simulink model "Autonomous_Driving"  (R2021a)
settings: Solver=ode2  StartTime=0.0  StopTime=inf  FixedStep=1/600  RelTol=1e-3  EnableMultiTasking=on
model workspace (MAT data in the model file):
  camera_rate : Simulink.Parameter (value not decoded)
  depth_rate : Simulink.Parameter (value not decoded)
symbols that are objects in the model workspace (value not decoded): camera_rate, depth_rate
undefined symbols (not defined in the file): gcbh, HIL, JPEG, qc_get_step_size, Video3D, video_display_show
libraries: quarc_library x32, simulink x15
(part 2 of 2)

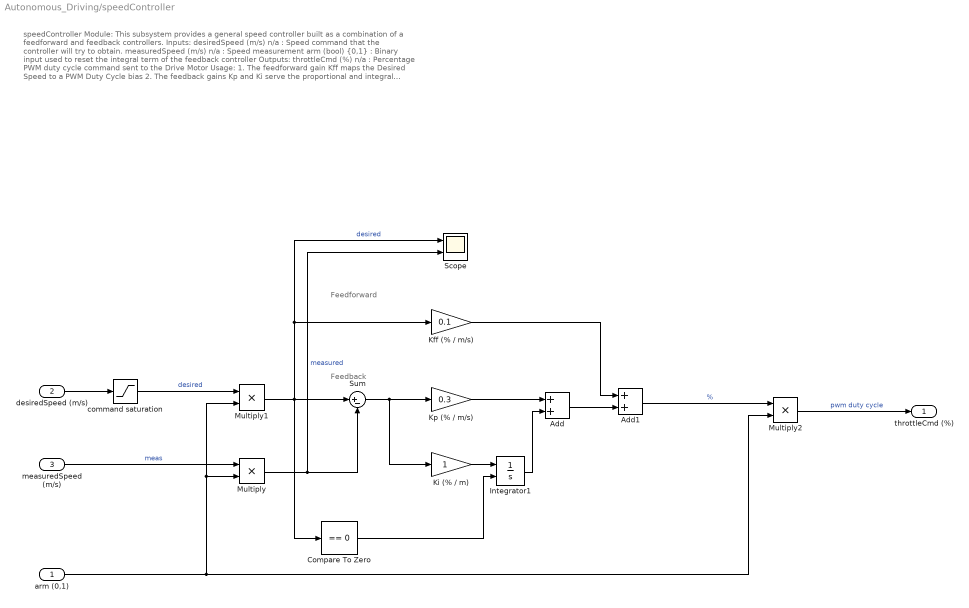
== system Autonomous_Driving/speedController ==
  note: Feedforward
  note: Feedback
  note: speedController Module:
      |
      | This subsystem provides a general speed controller built as a combination of a feedforward and feedback controllers.
      |
      | Inputs:
      | desiredSpeed (m/s) n/a : Speed command that the controller will try to obtain.
      | measuredSpeed (m/s) n/a : Speed measurement
      | arm (bool) {0,1} : Binary input used to reset the integral term of the feedback controller
      |
      | Outputs:
      | throttleCmd (%) n/a : Percentage PWM duty cycle command sent to the Drive Motor
      |
      | Usage:
      | 1. The feedforward gain Kff maps the Desired Speed to a PWM Duty Cycle bias
      | 2. The feedback gains Kp and Ki serve the proportional and integral terms to output corrections to the PWM Duty Cycle so as to regulate the desired speed.
  arm (0,1) : Inport
  desiredSpeed (m/s) : Inport  Port=2
  measuredSpeed (m/s) : Inport  Port=3
  Add : Sum
  Add1 : Sum
  Compare To Zero : simulink/Logic and Bit Operations/Compare To Zero  relop===  OutDataTypeStr=boolean
  Integrator1 : Integrator  ExternalReset=either  LimitOutput=on  UpperSaturationLimit=0.4  LowerSaturationLimit=-0.4
  Kff (% / m/s) : Gain  Gain=0.1
  "Ki (% / m) " : Gain
  Kp (% / m/s) : Gain  Gain=0.3
  Multiply : Product
  Multiply1 : Product
  Multiply2 : Product
  Scope : Scope  NumInputPorts=2
  Sum : Sum  Inputs=|+-
  command saturation : Saturate  UpperLimit=5  LowerLimit=-5
  throttleCmd (%) : Outport  VectorParamsAs1DForOutWhenUnconnected=off
  wires:
  command saturation/1 -> Multiply1/1  "desired"
  arm (0,1)/1 -> Multiply1/2, Multiply/2, Multiply2/2
  measuredSpeed (m/s)/1 -> Multiply/1  "meas"
  Multiply/1 -> Sum/2, Scope/2  "measured"
  Add/1 -> Add1/2
  Add1/1 -> Multiply2/1  "%"
  Multiply1/1 -> Compare To Zero/1, Sum/1, Kff (% / m/s)/1, Scope/1  "desired"
  Integrator1/1 -> Add/2
  Multiply2/1 -> throttleCmd (%)/1  "pwm duty cycle"
  Kp (% / m/s)/1 -> Add/1
  Compare To Zero/1 -> Integrator1/2
  Kff (% / m/s)/1 -> Add1/1
  Sum/1 -> "Ki (% / m) "/1, Kp (% / m/s)/1
  "Ki (% / m) "/1 -> Integrator1/1
  desiredSpeed (m/s)/1 -> command saturation/1

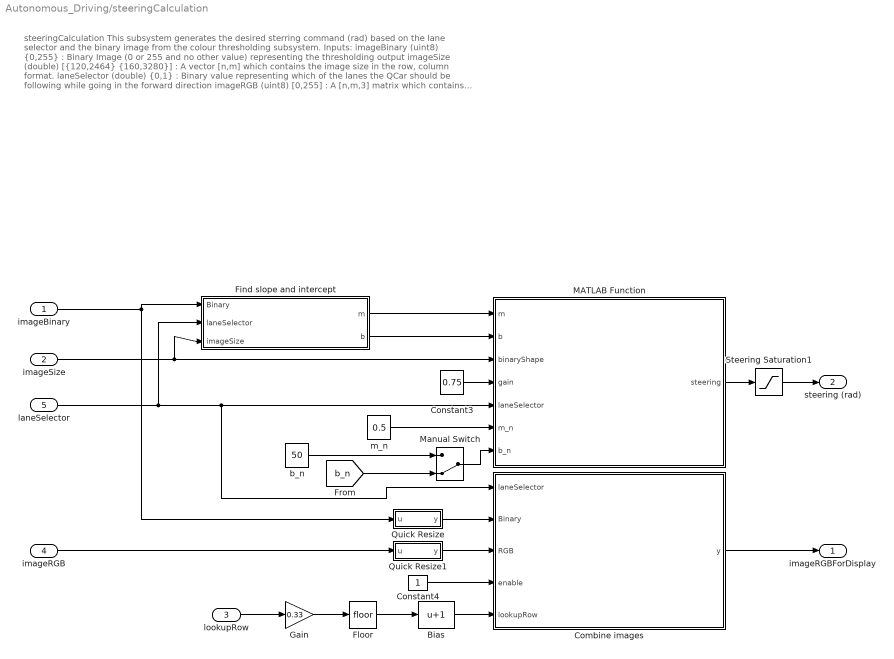
== system Autonomous_Driving/steeringCalculation ==
  note: steeringCalculation
      | This subsystem generates the desired sterring command (rad) based on the lane selector and the binary image from the colour thresholding subsystem.
      |
      | Inputs:
      | imageBinary (uint8) {0,255} : Binary Image (0 or 255 and no other value) representing the thresholding output
      | imageSize (double) [{120,2464} {160,3280}] : A vector [n,m] which contains the image size in the row, column format.
      | laneSelector (double) {0,1} : Binary value representing which of the lanes the QCar should be following while going in the forward direction
      | imageRGB (uint8) [0,255] : A [n,m,3] matrix which contains RGB values of an image in uint8 format
      |
      | Outputs:
      | steering (double) {-0.5,0.5} : Angle in rad representing the desired steering command based on the linearPolyFit
      | imageRGBForDisplay (uint8) {0,255} : A [n,m,3] matrix representing an RGB Image with mask of the lane currently being tracked
      |
      | Usage:
      |
      | This module can be used to generate a desired steering angle based on a thresheld image. A linear polygonal fit is used to generate a slope based on the equation y = mx+b whose slope and y intercept will define the steering angle commanded up to 0.5 (rad). The RGB image is a combination of the binary image holding information of the lane being followed, and a scaled version of the original RGB image.
  imageBinary : Inport
  imageSize : Inport  Port=2
  lookupRow : Inport  Port=3
  imageRGB : Inport  Port=4
  laneSelector : Inport  Port=5
  Bias : Bias  Bias=1
  Combine images : MATLAB Function  TreatAsAtomicUnit=on
  Constant3 : Constant  Value=0.75
  Constant4 : Constant
  Find slope and intercept : MATLAB Function  TreatAsAtomicUnit=on
  Floor : Rounding
  Gain : Gain  Gain=0.33
  MATLAB Function : MATLAB Function  TreatAsAtomicUnit=on
  Manual Switch : ManualSwitch  CurrentSetting=0
  Quick Resize : MATLAB Function  TreatAsAtomicUnit=on
  Quick Resize1 : MATLAB Function  TreatAsAtomicUnit=on
  Steering Saturation1 : Saturate
  b_n : Constant  Value=50
  m_n : Constant  Value=0.5
  imageRGBForDisplay : Outport  VectorParamsAs1DForOutWhenUnconnected=off
  steering (rad) : Outport  Port=2  VectorParamsAs1DForOutWhenUnconnected=off
  wires:
  Find slope and intercept/1(m) -> MATLAB Function/1(m)
  laneSelector/1 -> MATLAB Function/5(laneSelector), Combine images/1(laneSelector), Find slope and intercept/2(laneSelector)
  MATLAB Function/1(steering) -> Steering Saturation1/1
  Constant3/1 -> MATLAB Function/4(gain)
  imageBinary/1 -> Quick Resize/1(u), Find slope and intercept/1(Binary)
  Find slope and intercept/2(b) -> MATLAB Function/2(b)
  Constant4/1 -> Combine images/4(enable)
  Quick Resize/1(y) -> Combine images/2(Binary)
  Quick Resize1/1(y) -> Combine images/3(RGB)
  Combine images/1(y) -> imageRGBForDisplay/1
  imageRGB/1 -> Quick Resize1/1(u)
  Steering Saturation1/1 -> steering (rad)/1
  Gain/1 -> Floor/1
  imageSize/1 -> Find slope and intercept/3(imageSize), MATLAB Function/3(binaryShape)
  lookupRow/1 -> Gain/1
  Bias/1 -> Combine images/5(lookupRow)
  Floor/1 -> Bias/1
  b_n/1 -> Manual Switch/1
  Manual Switch/1 -> MATLAB Function/7(b_n)
  [b_n] -> Manual Switch/2
  m_n/1 -> MATLAB Function/6(m_n)

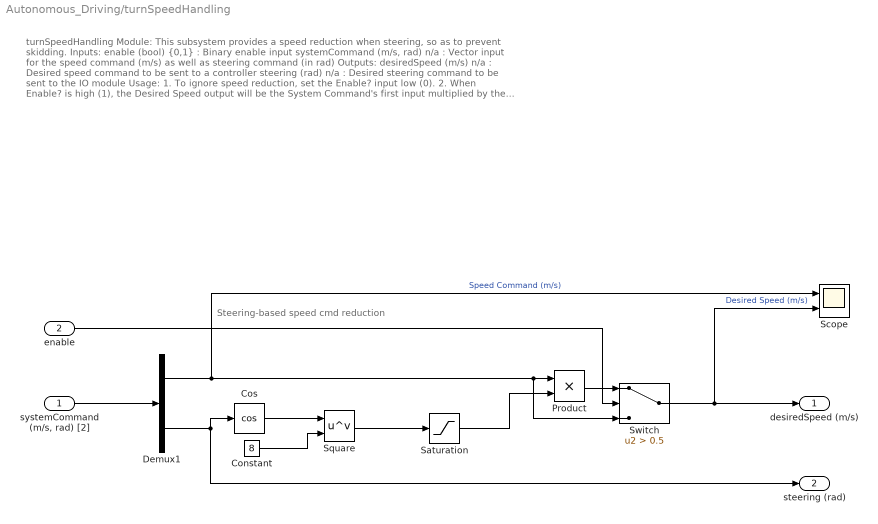
== system Autonomous_Driving/turnSpeedHandling ==
  note: turnSpeedHandling Module:
      |
      | This subsystem provides a speed reduction when steering, so as to prevent skidding.
      |
      | Inputs:
      | enable (bool) {0,1} : Binary enable input
      | systemCommand (m/s, rad) n/a : Vector input for the speed command (m/s) as well as steering command (in rad)
      |
      | Outputs:
      | desiredSpeed (m/s) n/a : Desired speed command to be sent to a controller
      | steering (rad) n/a : Desired steering command to be sent to the IO module
      |
      | Usage:
      | 1. To ignore speed reduction, set the Enable? input low (0).
      | 2. When Enable? is high (1), the Desired Speed output will be the System Command's first input multiplied by the cosine of the steering. Note that the lower limit of this reduction is set to 50% of the speed command input.
  note: Steering-based speed cmd reduction
  "systemCommand (m/s, rad) [2]" : Inport
  enable : Inport  Port=2
  Constant : Constant  Value=8
  Cos : Trigonometry  Operator=cos
  Demux1 : Demux  Outputs=2
  Product : Product
  Saturation : Saturate  UpperLimit=1  LowerLimit=0.5
  Scope : Scope  NumInputPorts=2
  Square : Math  Operator=pow  SignedPower=on  SaturateOnIntegerOverflow=on
  Switch : Switch  Criteria=u2 > Threshold  Threshold=0.5
  desiredSpeed (m/s) : Outport  VectorParamsAs1DForOutWhenUnconnected=off
  steering (rad) : Outport  Port=2  VectorParamsAs1DForOutWhenUnconnected=off
  wires:
  Cos/1 -> Square/1
  Switch/1 -> desiredSpeed (m/s)/1, Scope/2  "Desired Speed (m/s)"
  Product/1 -> Switch/1
  Saturation/1 -> Product/2
  Demux1/1 -> Product/1, Switch/3, Scope/1  "Speed Command (m/s)"
  "systemCommand (m/s, rad) [2]"/1 -> Demux1/1
  enable/1 -> Switch/2
  Constant/1 -> Square/2
  Demux1/2 -> steering (rad)/1, Cos/1
  Square/1 -> Saturation/1

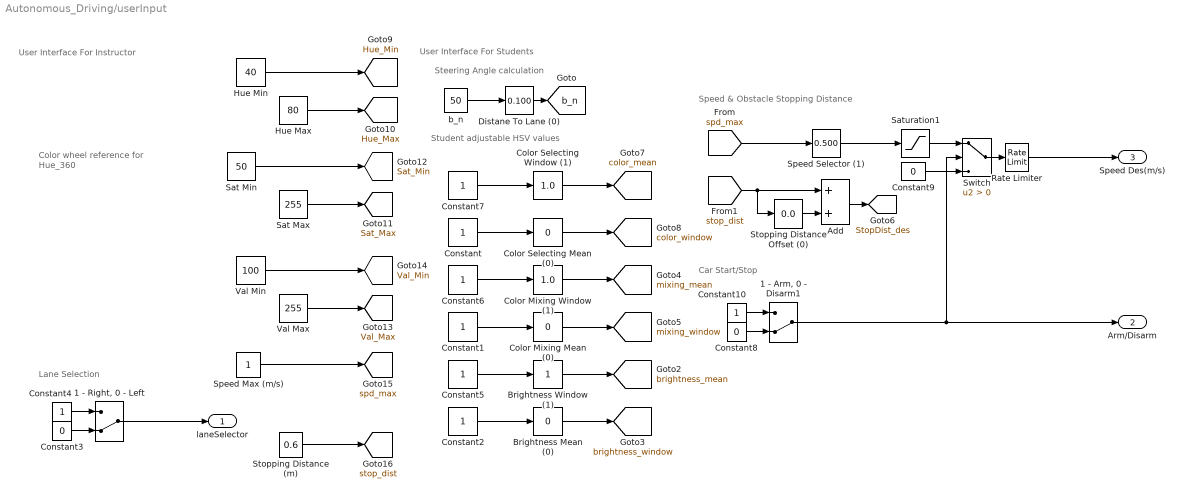
== system Autonomous_Driving/userInput ==
  note: User Interface For Instructor
  note: Student adjustable HSV values
  note: Lane Selection
  note: Car Start/Stop
  note: Steering Angle calculation
  note: User Interface For Students
  note: Speed & Obstacle Stopping Distance
  note: Color wheel
      | reference
      | for Hue_360
  "1 - Arm, 0 - Disarm1" : ManualSwitch  CurrentSetting=0
  "1 - Right, 0 - Left" : ManualSwitch  CurrentSetting=0
  Add : Sum
  Brightness Mean (0) : simulink/Math Operations/Slider Gain  gain=0  low=-1  high=1
  Brightness Window (1) : simulink/Math Operations/Slider Gain  gain=1  low=0  high=1
  Color Mixing Mean (0) : simulink/Math Operations/Slider Gain  gain=0  low=-1  high=1
  Color Mixing Window (1) : simulink/Math Operations/Slider Gain  gain=1.0  low=0  high=1
  Color Selecting Mean (0) : simulink/Math Operations/Slider Gain  gain=0  low=-1  high=1
  Color Selecting Window (1) : simulink/Math Operations/Slider Gain  gain=1.0  low=0  high=1
  Constant{,1..2,4..7,10} (8 alike) : Constant
  Constant3 : Constant  Value=0
  Constant8 : Constant  Value=0
  Constant9 : Constant  Value=0
  "Distane To Lane (0) " : simulink/Math Operations/Slider Gain  gain=0.100  low=0  high=1
  Hue Max : Constant  Value=80
  Hue Min : Constant  Value=40
  Rate Limiter : RateLimiter  FallingSlewLimit=-Inf  SampleTimeMode=inherited
  Sat Max : Constant  Value=255
  Sat Min : Constant  Value=50
  Saturation1 : Saturate  UpperLimit=1  LowerLimit=0
  Speed Max (m/s) : Constant
  Speed Selector (1) : simulink/Math Operations/Slider Gain  gain=0.500  low=0  high=1
  Stopping Distance (m) : Constant  Value=0.6
  Stopping Distance Offset (0) : simulink/Math Operations/Slider Gain  gain=0.0  low=0  high=1
  Switch : Switch  Criteria=u2 > Threshold
  Val Max : Constant  Value=255
  Val Min : Constant  Value=100
  b_n : Constant  Value=50
  laneSelector : Outport  VectorParamsAs1DForOutWhenUnconnected=off
  Arm/Disarm : Outport  Port=2  VectorParamsAs1DForOutWhenUnconnected=off
  Speed Des(m/s) : Outport  Port=3  VectorParamsAs1DForOutWhenUnconnected=off
  tag scope: Hue_Max=global, Hue_Min=global, Sat_Max=global, Sat_Min=global, StopDist_des=global, Val_Max=global, Val_Min=global, b_n=global, brightness_mean=global, brightness_window=global, color_mean=global, color_window=global, mixing_mean=global, mixing_window=global, spd_max=global, stop_dist=global
  wires:
  Constant3/1 -> "1 - Right, 0 - Left"/2
  "1 - Arm, 0 - Disarm1"/1 -> Switch/2, Arm/Disarm/1
  b_n/1 -> "Distane To Lane (0) "/1
  Constant4/1 -> "1 - Right, 0 - Left"/1
  Switch/1 -> Rate Limiter/1
  Constant9/1 -> Switch/3
  [spd_max] -> Speed Selector (1)/1
  Saturation1/1 -> Switch/1
  Constant10/1 -> "1 - Arm, 0 - Disarm1"/1
  "1 - Right, 0 - Left"/1 -> laneSelector/1
  Rate Limiter/1 -> Speed Des(m/s)/1
  Constant8/1 -> "1 - Arm, 0 - Disarm1"/2
  "Distane To Lane (0) "/1 -> [b_n]
  Color Mixing Window (1)/1 -> [mixing_mean]
  Constant/1 -> Color Selecting Mean (0)/1
  Constant2/1 -> Brightness Mean (0)/1
  Constant5/1 -> Brightness Window (1)/1
  Constant1/1 -> Color Mixing Mean (0)/1
  Color Selecting Mean (0)/1 -> [color_window]
  Brightness Window (1)/1 -> [brightness_mean]
  Color Selecting Window (1)/1 -> [color_mean]
  Brightness Mean (0)/1 -> [brightness_window]
  Color Mixing Mean (0)/1 -> [mixing_window]
  Constant6/1 -> Color Mixing Window (1)/1
  Constant7/1 -> Color Selecting Window (1)/1
  Hue Min/1 -> [Hue_Min]
  Sat Min/1 -> [Sat_Min]
  Val Min/1 -> [Val_Min]
  Hue Max/1 -> [Hue_Max]
  Sat Max/1 -> [Sat_Max]
  Val Max/1 -> [Val_Max]
  Speed Selector (1)/1 -> Saturation1/1
  Speed Max (m/s)/1 -> [spd_max]
  Stopping Distance (m)/1 -> [stop_dist]
  [stop_dist] -> Stopping Distance Offset (0)/1, Add/1
  Stopping Distance Offset (0)/1 -> Add/2
  Add/1 -> [StopDist_des]

== system Autonomous_Driving/Display Depth/Depth Camera Information ==
  In1 : Inport
  Channel : quarc_library/Signal Routing/Channel  channel=0  buffer_size=1
  Image Compress : quarc_library/Image Processing/Generic/Image Compress  algorithm=JPEG  source=Internal dialog parameter  quality=quality  output_dim=-1
  Video Display : quarc_library/Multimedia/Video Display  Tag=Autonomous_Driving/Display Depth/Depth Camera Information/Video Display  sample_time=sample_time  use_hardware=on
  wires:
  Image Compress/1 -> Channel/1
  In1/1 -> Image Compress/1
  Channel/1 -> Video Display/1

== system Autonomous_Driving/Display RGB/RGB Image Processed ==
  In1 : Inport
  Channel : quarc_library/Signal Routing/Channel  channel=1  buffer_size=1
  Image Compress : quarc_library/Image Processing/Generic/Image Compress  algorithm=JPEG  source=Internal dialog parameter  quality=quality  output_dim=-1
  Video Display : quarc_library/Multimedia/Video Display  Tag=Autonomous_Driving/Display RGB/RGB Image Processed/Video Display  sample_time=sample_time  use_hardware=on
  wires:
  Image Compress/1 -> Channel/1
  In1/1 -> Image Compress/1
  Channel/1 -> Video Display/1

== system Autonomous_Driving/RGB Image Pre-Proccessing/RGB Image No Threshold ==
  In1 : Inport
  Channel : quarc_library/Signal Routing/Channel  channel=2  buffer_size=1
  Image Compress : quarc_library/Image Processing/Generic/Image Compress  algorithm=JPEG  source=Internal dialog parameter  quality=quality  output_dim=-1
  Video Display : quarc_library/Multimedia/Video Display  Tag="Autonomous_Driving/RGB Image  Pre-Proccessing/RGB Image No Threshold/Video Display"  sample_time=sample_time  use_hardware=on
  wires:
  Channel/1 -> Video Display/1
  In1/1 -> Image Compress/1
  Image Compress/1 -> Channel/1

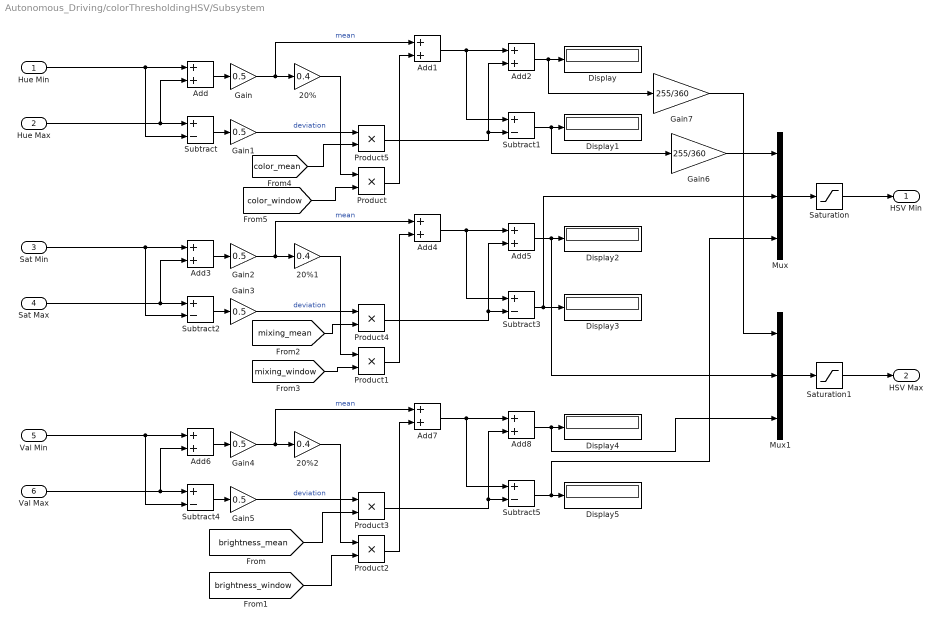
== system Autonomous_Driving/colorThresholdingHSV/Subsystem ==
  Hue Min : Inport
  Hue Max : Inport  Port=2
  Sat Min : Inport  Port=3
  Sat Max : Inport  Port=4
  Val Min : Inport  Port=5
  Val Max : Inport  Port=6
  20% : Gain  Gain=0.4
  20%1 : Gain  Gain=0.4
  20%2 : Gain  Gain=0.4
  Add{,1..8} (9 alike) : Sum
  Display{,1..5} (6 alike) : Display
  Gain{,1..5} (6 alike) : Gain  Gain=0.5
  Gain6 : Gain  Gain=255/360
  Gain7 : Gain  Gain=255/360
  Mux : Mux  Inputs=3
  Mux1 : Mux  Inputs=3
  Product{,1..5} (6 alike) : Product
  Saturation : Saturate  UpperLimit=[255 255 255]  LowerLimit=[0 0 0]
  Saturation1 : Saturate  UpperLimit=[255 255 255]  LowerLimit=[0 0 0]
  Subtract{,1..5} (6 alike) : Sum  Inputs=+-
  HSV Min : Outport  VectorParamsAs1DForOutWhenUnconnected=off
  HSV Max : Outport  Port=2  VectorParamsAs1DForOutWhenUnconnected=off
  wires:
  Product1/1 -> Add4/2
  Val Min/1 -> Add6/1, Subtract4/2
  Mux/1 -> Saturation/1
  Subtract1/1 -> Gain6/1, Display1/1
  Subtract4/1 -> Gain5/1
  Add1/1 -> Subtract1/1, Add2/1
  Product3/1 -> Add8/2, Subtract5/2
  Product2/1 -> Add7/2
  Gain4/1 -> 20%2/1, Add7/1  "mean"
  Add2/1 -> Gain7/1, Display/1
  Subtract3/1 -> Mux/2, Display3/1
  Subtract5/1 -> Mux/3, Display5/1
  Gain/1 -> 20%/1, Add1/1  "mean"
  Sat Min/1 -> Subtract2/2, Add3/1
  Subtract2/1 -> Gain3/1
  Product5/1 -> Add2/2, Subtract1/2
  Gain5/1 -> Product3/1  "deviation"
  Add5/1 -> Mux1/2, Display2/1
  Gain2/1 -> Add4/1, 20%1/1  "mean"
  Add8/1 -> Mux1/3, Display4/1
  Product/1 -> Add1/2
  Subtract/1 -> Gain1/1
  Product4/1 -> Subtract3/2, Add5/2
  Add4/1 -> Add5/1, Subtract3/1
  Add7/1 -> Subtract5/1, Add8/1
  Sat Max/1 -> Subtract2/1, Add3/2
  20%1/1 -> Product1/1
  [brightness_mean] -> Product3/2
  Mux1/1 -> Saturation1/1
  Add3/1 -> Gain2/1
  [mixing_mean] -> Product4/2
  Hue Min/1 -> Add/1, Subtract/2
  Hue Max/1 -> Add/2, Subtract/1
  Gain3/1 -> Product4/1  "deviation"
  Val Max/1 -> Add6/2, Subtract4/1
  20%2/1 -> Product2/1
  Add6/1 -> Gain4/1
  [color_window] -> Product/2
  [color_mean] -> Product5/2
  20%/1 -> Product/1
  Add/1 -> Gain/1
  Gain1/1 -> Product5/1  "deviation"
  [mixing_window] -> Product1/2
  [brightness_window] -> Product2/2
  Saturation/1 -> HSV Min/1
  Saturation1/1 -> HSV Max/1
  Gain6/1 -> Mux/1
  Gain7/1 -> Mux1/1

== matlab function Autonomous_Driving/MATLAB Function ==
  data: imageRGB input; imageToThreshold output; laneSelector input; lookupRow input; imageSize output
function [imageToThreshold, imageSize]  = imageSelector(imageRGB, laneSelector, lookupRow)

[ROW, COL, ~] = size(imageRGB);
% imageToThreshold = uint8(zeros(ROW/2+1,COL/3,3));
if laneSelector
    imageToThreshold = imageRGB(ROW/2+1:ROW, COL*(2/3) + 1:COL, :);
else
    imageToThreshold = imageRGB(ROW/2+1:ROW, 1:COL/3, :);
end
imageToThreshold(1: ROW/2 - (ROW - lookupRow + 1),:,:) = 0;
imageSize = [ROW - lookupRow + 1, COL/3];

== matlab function Autonomous_Driving/obstacleDetection/Draw Lines Module ==
  data: img_in input; img_out output; pts input; color input
function img_out = drawLines(img_in, pts, color)

% Draw lines connecting the points using the provided color

% Inputs:
% img_in    : Input RGB Image (size = m by n)
% pts       : p x-y pairs of points (px) where markers are to be drawn
% color     : 1x3 matrix of RGB color values for each marker

% Outputs:
% img_out   : Output RGB Image with the markers drawn in (size = m by n)

%% Initialization
if size(img_in, 3) == 3
    img_out = img_in;
elseif size(img_in, 3) == 1
    img_out = cat(3, img_in, img_in, img_in);
end

[p, ~] = size(pts); % determine the number of points

%% Draw the lines
    for i = 1:p-1
        % determine the max(rows_difference, col_difference) between two
        % points
        itr = max(abs(pts(i,1) - pts(i+1,1)), abs(pts(i,2) - pts(i+1,2)));
        
        % generate linear spaces of row and col values between the pts
        row_vec = round(linspace(pts(i,1), pts(i+1,1), itr));
        col_vec = round(linspace(pts(i,2), pts(i+1,2), itr));
        
        % iterate through the values and shade them right

        for j = 1:itr
            img_out(row_vec(j), col_vec(j),1) = color(1);
            img_out(row_vec(j), col_vec(j),2) = color(2);
            img_out(row_vec(j), col_vec(j),3) = color(3);
        end
    end
end

== matlab function Autonomous_Driving/steeringCalculation/Find slope and intercept ==
  data: Binary input; m output; b output; laneSelector input; imageSize input
function [m, b] = linearPolyFit(Binary, laneSelector, imageSize)

% find the shape of the incoming image
[ROW, ~] = size(Binary);

% find row, col pairs of points where pixel value is bright
[rows, cols] = find(Binary(ROW - imageSize(1) + 1:end, :) > 0);

% x is coloumns, y is max_row - rows
if laneSelector
    x = imageSize(2) - cols;
else
    x = cols;
end

y = imageSize(1) - rows;

% fit a linear polynomial to the points and grab slope, intercept
% result = polyfit(x(idx), y(idx), 1);
result = polyfit(x, y, 1);
m = result(1); 
b = result(2);

== matlab function Autonomous_Driving/steeringCalculation/MATLAB Function ==
  data: m input; steering output; b input; binaryShape input; gain input; laneSelector input; m_n input; b_n input
function steering = fcn(m, b, binaryShape, gain, laneSelector, m_n, b_n)
 
% y = mx + b

current_x = (binaryShape(1) - b)/m;
nominal_x = (binaryShape(1) - b_n)/m_n;
if laneSelector
    steering = -gain*(nominal_x - current_x)/binaryShape(2);
else
    steering = gain*(nominal_x - current_x)/binaryShape(2);
end

== matlab function Autonomous_Driving/steeringCalculation/Quick Resize ==
  data: u input; y output
function y = quickResize(u)

scale = 3;
    if length(size(u)) == 3
        y = u(1:scale:end, 1:scale:end, :);
    else
        y = u(1:scale:end, 1:scale:end);
    end

end

== matlab function Autonomous_Driving/steeringCalculation/Combine images ==
  data: laneSelector input; Binary input; RGB input; y output size=[137,274,3]; enable input; lookupRow input
function y = laneMask(laneSelector, Binary, RGB, enable, lookupRow)

y = RGB;
[ROW, COL, ~] = size(y);
[binRow, ~] = size(Binary);
binarySection = Binary(binRow-(length(lookupRow:ROW))+1:binRow,:);
if enable
    if laneSelector
        section = RGB(lookupRow:ROW, COL*(2/3) + 1:COL, :);
        y(lookupRow:ROW, COL*(2/3) + 1:COL, 1) = ((255 - binarySection)/255).*section(:,:,1) + (binarySection).*section(:, :, 1);
        y(lookupRow:ROW, COL*(2/3) + 1:COL, 2) = ((255 - binarySection)/255).*section(:,:,2);
        y(lookupRow:ROW, COL*(2/3) + 1:COL, 3) = ((255 - binarySection)/255).*section(:,:,3);
    else
        section = RGB(lookupRow:ROW, 1:COL/3, :);
        y(lookupRow:ROW, 1:COL/3, 1) = ((255 - binarySection)/255).*section(:,:,1) + (binarySection).*section(:, :, 1);
        y(lookupRow:ROW, 1:COL/3, 2) = ((255 - binarySection)/255).*section(:,:,2);
        y(lookupRow:ROW, 1:COL/3, 3) = ((255 - binarySection)/255).*section(:,:,3);
    end
end

== matlab function Autonomous_Driving/obstacleDetection/MATLAB Function ==
  data: depth input; y output; minDistance input; maxDistance input
function y = calculateDistance(depth, minDistance, maxDistance)

% This function drops depth data when outside the minDistance:maxDistance
% bounds and then averages the result. 

% u_flat = reshape(depth, 1, []);
% u_flat(u_flat < minDistance) = [];
% u_flat(u_flat > maxDistance) = [];
% y = mean(mean(u_flat));


u_flat = depth(depth <maxDistance);

u_flat  = depth(u_flat>minDistance);

y = mean(u_flat);

== matlab function Autonomous_Driving/obstacleDetection/Steering based image subselector ==
  data: pts output; depth input; region output; steering input
function [pts, region] = drawBox(depth, steering)
% Input: 640 x 360
mark = 320 - (steering*260/0.5);
starting_index = mark+1-60;
region = double(depth(121:240, starting_index : starting_index + 119));
pts = [ 101, mark+1-60; 101, mark+60; 220, mark+60; 220, mark+1-60; 101, mark+1-60];

== matlab function Autonomous_Driving/steeringCalculation/Quick Resize1 ==
  data: u input; y output
function y = quickResize(u)

scale = 3;
    if length(size(u)) == 3
        y = u(1:scale:end, 1:scale:end, :);
    else
        y = u(1:scale:end, 1:scale:end);
    end

end

== matlab function Autonomous_Driving/automatedDriving/MATLAB Function ==
  data: obstacle_distance input; speed_cmd output; stop_distance input; nominal_tracking_distance input; nominal_speed input
function speed_cmd = adaptive_cruise_control(obstacle_distance, stop_distance, nominal_tracking_distance, nominal_speed)

speed_cmd = nominal_speed;

if obstacle_distance < stop_distance
    speed_cmd = 0;
    
elseif obstacle_distance < nominal_tracking_distance
    speed_cmd = nominal_speed/(nominal_tracking_distance-stop_distance)*obstacle_distance...
              - nominal_speed/(nominal_tracking_distance-stop_distance)*stop_distance;

end
